simulink model "SimulModeloDinamico"  (R2015a)
settings: Solver=ode4  StartTime=0.0  StopTime=10.0  FixedStep=.001  RelTol=1e-3
libraries: dspinverses x1
settings Model: Creator=Sala6  LastModifiedBy=Sala1

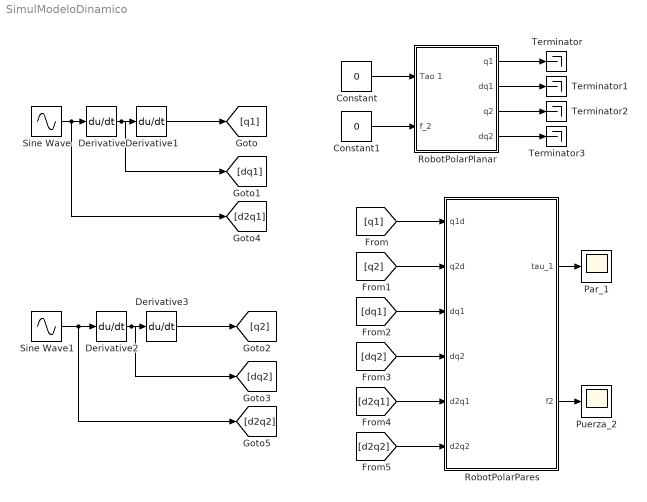
== system SimulModeloDinamico ==
  Constant : Constant  Value=0
  Constant1 : Constant  Value=0
  Derivative{,1..3} (4 alike) : Derivative
  "Par_1 " : Scope
  Puerza_2 : Scope
  RobotPolarPares : Subsystem  mask{m1=.2, m2=.1, l1=.15, lc1=.075, lc2=.05, I1z=.002, I2z=.001, g=9.81, q1_0=pi/3, dq1_0=0, q2_0=.15, dq2_0=0}
      mask prompts: m1 "Masa Eslabon1"; m2 "Masa Eslabon2"; l1 "Longitud Eslabon1"; lc1 "Longitud al Centro de Masa 1"; lc2 "Longitud al Centro de Masa 1"; I1z "Momento de Inercia Eslabon 1"; I2z "Momento de Inercia Eslabon 2"; g "Constante de Gravedad (g)"; q1_0 "Posicion inicial eslabon 1"; dq1_0 "Velocidad inicial eslabon 1"; q2_0 "Posicion inicial eslabon 2"; dq2_0 "Velocidad inicial eslabon 1"
  RobotPolarPlanar : Subsystem  mask{m1=.2, m2=.1, l1=.15, lc1=.075, lc2=.05, I1z=.002, I2z=.001, g=9.81, q1_0=pi/3, dq1_0=0, q2_0=.15, dq2_0=0}
      mask prompts: m1 "Masa Eslabon1"; m2 "Masa Eslabon2"; l1 "Longitud Eslabon1"; lc1 "Longitud al Centro de Masa 1"; lc2 "Longitud al Centro de Masa 1"; I1z "Momento de Inercia Eslabon 1"; I2z "Momento de Inercia Eslabon 2"; g "Constante de Gravedad (g)"; q1_0 "Posicion inicial eslabon 1"; dq1_0 "Velocidad inicial eslabon 1"; q2_0 "Posicion inicial eslabon 2"; dq2_0 "Velocidad inicial eslabon 1"
  Sine Wave : Sin  Amplitude=pi/2  Frequency=4*pi  SampleTime=0
  Sine Wave1 : Sin  Amplitude=.1  Frequency=2*pi  SampleTime=0
  Terminator{,1..3} (4 alike) : Terminator
  wires:
  Sine Wave/1 -> [d2q1], Derivative/1
  Derivative/1 -> [dq1], Derivative1/1
  Derivative1/1 -> [q1]
  Sine Wave1/1 -> [d2q2], Derivative2/1
  Derivative2/1 -> Derivative3/1, [dq2]
  Derivative3/1 -> [q2]
  [q1] -> RobotPolarPares/1(q1d)
  [q2] -> RobotPolarPares/2(q2d)
  [dq1] -> RobotPolarPares/3(dq1)
  [dq2] -> RobotPolarPares/4(dq2)
  [d2q1] -> RobotPolarPares/5(d2q1)
  [d2q2] -> RobotPolarPares/6(d2q2)
  RobotPolarPares/1(tau_1) -> "Par_1 "/1
  RobotPolarPares/2(f2) -> Puerza_2/1
  RobotPolarPlanar/2(dq1) -> Terminator1/1
  RobotPolarPlanar/1(q1) -> Terminator/1
  RobotPolarPlanar/3(q2) -> Terminator2/1
  RobotPolarPlanar/4(dq2) -> Terminator3/1
  Constant/1 -> RobotPolarPlanar/1("Tao 1 ")
  Constant1/1 -> RobotPolarPlanar/2("f_2 ")

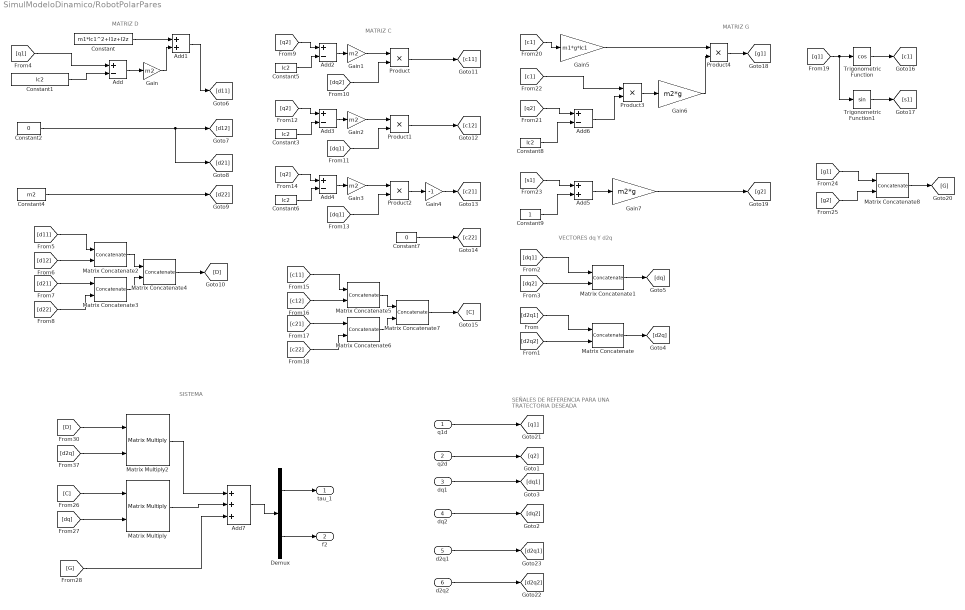
== system SimulModeloDinamico/RobotPolarPares ==
  note: SISTEMA
  note: SEÑALES DE REFERENCIA PARA UNA TRATECTORIA DESEADA
  note: MATRIZ D
  note: MATRIZ C
  note: VECTORES dq Y d2q
  note: MATRIZ G
  q1d : Inport
  q2d : Inport  Port=2
  dq1 : Inport  Port=3
  dq2 : Inport  Port=4
  d2q1 : Inport  Port=5
  d2q2 : Inport  Port=6
  Add{,2..4,6} (5 alike) : Sum  Inputs=+-
  Add1 : Sum
  Add5 : Sum
  Add7 : Sum  Inputs=+++
  Constant : Constant  Value=m1*lc1^2+I1z+I2z
  Constant{1,3,5..6,8} (5 alike) : Constant  Value=lc2
  Constant2 : Constant  Value=0
  Constant4 : Constant  Value=m2
  Constant7 : Constant  Value=0
  Constant9 : Constant
  Demux : Demux  Outputs=2
  Gain{,1..3} (4 alike) : Gain  Gain=m2
  Gain4 : Gain  Gain=-1
  Gain5 : Gain  Gain=m1*g*lc1
  Gain6 : Gain  Gain=m2*g
  Gain7 : Gain  Gain=m2*g
  Matrix Concatenate{,1,4,7..8} (5 alike) : Concatenate  Mode=Multidimensional array
  Matrix Concatenate{2..3,5..6} (4 alike) : Concatenate  Mode=Multidimensional array  ConcatenateDimension=2
  Matrix Multiply : Product  Multiplication=Matrix(*)
  Matrix Multiply2 : Product  Multiplication=Matrix(*)
  Product{,1..4} (5 alike) : Product
  Trigonometric Function : Trigonometry  Operator=cos
  Trigonometric Function1 : Trigonometry
  tau_1 : Outport
  f2 : Outport  Port=2
  wires:
  Demux/2 -> f2/1
  Demux/1 -> tau_1/1
  Add7/1 -> Demux/1
  [dq] -> Matrix Multiply/2
  [C] -> Matrix Multiply/1
  q1d/1 -> [q1]
  q2d/1 -> [q2]
  Matrix Concatenate8/1 -> [G]
  [g2] -> Matrix Concatenate8/2
  [g1] -> Matrix Concatenate8/1
  Gain7/1 -> [g2]
  Add5/1 -> Gain7/1
  Constant9/1 -> Add5/2
  [s1] -> Add5/1
  Product4/1 -> [g1]
  Gain6/1 -> Product4/2
  Gain5/1 -> Product4/1
  Product3/1 -> Gain6/1
  Add6/1 -> Product3/2
  [c1] -> Product3/1
  Constant8/1 -> Add6/2
  [q2] -> Add6/1
  [c1] -> Gain5/1
  Trigonometric Function1/1 -> [s1]
  Trigonometric Function/1 -> [c1]
  [q1] -> Trigonometric Function/1, Trigonometric Function1/1
  Matrix Concatenate6/1 -> Matrix Concatenate7/2
  Matrix Concatenate5/1 -> Matrix Concatenate7/1
  [c12] -> Matrix Concatenate5/2
  [c22] -> Matrix Concatenate6/2
  [c21] -> Matrix Concatenate6/1
  Matrix Concatenate7/1 -> [C]
  [c11] -> Matrix Concatenate5/1
  Constant7/1 -> [c22]
  Gain4/1 -> [c21]
  Product2/1 -> Gain4/1
  [dq1] -> Product2/2
  Gain3/1 -> Product2/1
  Add4/1 -> Gain3/1
  Constant6/1 -> Add4/2
  [q2] -> Add4/1
  Product1/1 -> [c12]
  [dq1] -> Product1/2
  Gain2/1 -> Product1/1
  Add3/1 -> Gain2/1
  Constant3/1 -> Add3/2
  [q2] -> Add3/1
  Product/1 -> [c11]
  [dq2] -> Product/2
  Gain1/1 -> Product/1
  Add2/1 -> Gain1/1
  Constant5/1 -> Add2/2
  [q2] -> Add2/1
  Matrix Concatenate3/1 -> Matrix Concatenate4/2
  Matrix Concatenate2/1 -> Matrix Concatenate4/1
  [d12] -> Matrix Concatenate2/2
  [d22] -> Matrix Concatenate3/2
  [d21] -> Matrix Concatenate3/1
  Matrix Concatenate4/1 -> [D]
  [d11] -> Matrix Concatenate2/1
  Constant4/1 -> [d22]
  Constant2/1 -> [d12], [d21]
  Add1/1 -> [d11]
  Gain/1 -> Add1/2
  Constant/1 -> Add1/1
  Add/1 -> Gain/1
  Constant1/1 -> Add/2
  [q1] -> Add/1
  Matrix Concatenate1/1 -> [dq]
  Matrix Concatenate/1 -> [d2q]
  [dq2] -> Matrix Concatenate1/2
  [dq1] -> Matrix Concatenate1/1
  [d2q2] -> Matrix Concatenate/2
  [d2q1] -> Matrix Concatenate/1
  [d2q] -> Matrix Multiply2/2
  [D] -> Matrix Multiply2/1
  Matrix Multiply2/1 -> Add7/1
  Matrix Multiply/1 -> Add7/2
  [G] -> Add7/3
  dq1/1 -> [dq1]
  dq2/1 -> [dq2]
  d2q1/1 -> [d2q1]
  d2q2/1 -> [d2q2]

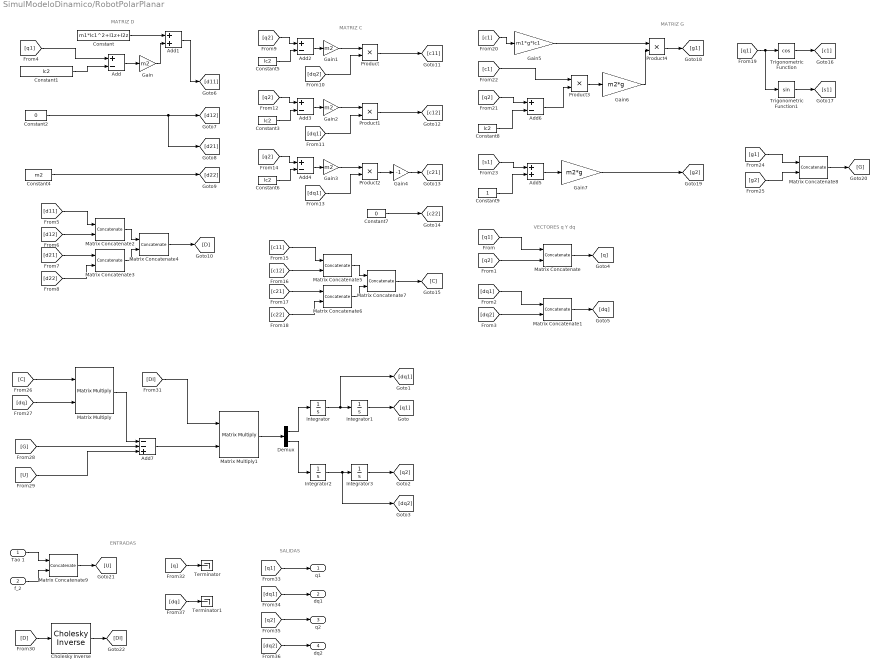
== system SimulModeloDinamico/RobotPolarPlanar ==
  note: ENTRADAS
  note: SALIDAS
  note: MATRIZ G
  note: VECTORES q Y dq
  note: MATRIZ C
  note: MATRIZ D
  "Tao 1 " : Inport
  "f_2 " : Inport  Port=2
  Add{,2..4,6} (5 alike) : Sum  Inputs=+-
  Add1 : Sum
  Add5 : Sum
  Add7 : Sum  Inputs=--+
  Cholesky Inverse : dspinverses/Cholesky Inverse  errmode=Warning
  Constant : Constant  Value=m1*lc1^2+I1z+I2z
  Constant{1,3,5..6,8} (5 alike) : Constant  Value=lc2
  Constant2 : Constant  Value=0
  Constant4 : Constant  Value=m2
  Constant7 : Constant  Value=0
  Constant9 : Constant
  Demux : Demux  Outputs=2
  Gain{,1..3} (4 alike) : Gain  Gain=m2
  Gain4 : Gain  Gain=-1
  Gain5 : Gain  Gain=m1*g*lc1
  Gain6 : Gain  Gain=m2*g
  Gain7 : Gain  Gain=m2*g
  Integrator : Integrator  InitialCondition=dq1_0
  Integrator1 : Integrator  InitialCondition=q1_0
  Integrator2 : Integrator  InitialCondition=dq2_0
  Integrator3 : Integrator  InitialCondition=q2_0
  Matrix Concatenate{,1,4,7..9} (6 alike) : Concatenate  Mode=Multidimensional array
  Matrix Concatenate{2..3,5..6} (4 alike) : Concatenate  Mode=Multidimensional array  ConcatenateDimension=2
  Matrix Multiply : Product  Multiplication=Matrix(*)
  Matrix Multiply1 : Product  Multiplication=Matrix(*)
  Product{,1..4} (5 alike) : Product
  Terminator : Terminator
  Terminator1 : Terminator
  Trigonometric Function : Trigonometry  Operator=cos
  Trigonometric Function1 : Trigonometry
  q1 : Outport
  dq1 : Outport  Port=2
  q2 : Outport  Port=3
  dq2 : Outport  Port=4
  wires:
  [q1] -> q1/1
  [dq1] -> dq1/1
  [q2] -> q2/1
  Integrator/1 -> [dq1], Integrator1/1
  Integrator2/1 -> [dq2], Integrator3/1
  Integrator1/1 -> [q1]
  Integrator3/1 -> [q2]
  [q1] -> Matrix Concatenate/1
  [q2] -> Matrix Concatenate/2
  [dq1] -> Matrix Concatenate1/1
  [dq2] -> Matrix Concatenate1/2
  Matrix Concatenate/1 -> [q]
  Matrix Concatenate1/1 -> [dq]
  [q1] -> Add/1
  Constant1/1 -> Add/2
  Add/1 -> Gain/1
  Constant/1 -> Add1/1
  Gain/1 -> Add1/2
  Add1/1 -> [d11]
  Constant2/1 -> [d21], [d12]
  Constant4/1 -> [d22]
  [d11] -> Matrix Concatenate2/1
  Matrix Concatenate4/1 -> [D]
  [d21] -> Matrix Concatenate3/1
  [d22] -> Matrix Concatenate3/2
  [d12] -> Matrix Concatenate2/2
  Matrix Concatenate2/1 -> Matrix Concatenate4/1
  Matrix Concatenate3/1 -> Matrix Concatenate4/2
  [q2] -> Add2/1
  Constant5/1 -> Add2/2
  Add2/1 -> Gain1/1
  Gain1/1 -> Product/1
  [dq2] -> Product/2
  Product/1 -> [c11]
  [q2] -> Add3/1
  Constant3/1 -> Add3/2
  Add3/1 -> Gain2/1
  Gain2/1 -> Product1/1
  [dq1] -> Product1/2
  Product1/1 -> [c12]
  [q2] -> Add4/1
  Constant6/1 -> Add4/2
  Add4/1 -> Gain3/1
  Gain3/1 -> Product2/1
  [dq1] -> Product2/2
  Product2/1 -> Gain4/1
  Gain4/1 -> [c21]
  Constant7/1 -> [c22]
  [c11] -> Matrix Concatenate5/1
  Matrix Concatenate7/1 -> [C]
  [c21] -> Matrix Concatenate6/1
  [c22] -> Matrix Concatenate6/2
  [c12] -> Matrix Concatenate5/2
  Matrix Concatenate5/1 -> Matrix Concatenate7/1
  Matrix Concatenate6/1 -> Matrix Concatenate7/2
  [q1] -> Trigonometric Function1/1, Trigonometric Function/1
  Trigonometric Function/1 -> [c1]
  Trigonometric Function1/1 -> [s1]
  [c1] -> Gain5/1
  [q2] -> Add6/1
  Constant8/1 -> Add6/2
  [c1] -> Product3/1
  Add6/1 -> Product3/2
  Product3/1 -> Gain6/1
  Gain5/1 -> Product4/1
  Gain6/1 -> Product4/2
  Product4/1 -> [g1]
  [s1] -> Add5/1
  Constant9/1 -> Add5/2
  Add5/1 -> Gain7/1
  Gain7/1 -> [g2]
  [g1] -> Matrix Concatenate8/1
  [g2] -> Matrix Concatenate8/2
  Matrix Concatenate8/1 -> [G]
  "Tao 1 "/1 -> Matrix Concatenate9/1
  "f_2 "/1 -> Matrix Concatenate9/2
  Matrix Concatenate9/1 -> [U]
  [C] -> Matrix Multiply/1
  [dq] -> Matrix Multiply/2
  Matrix Multiply/1 -> Add7/1
  [G] -> Add7/2
  [U] -> Add7/3
  [D] -> Cholesky Inverse/1
  Cholesky Inverse/1 -> [DI]
  Add7/1 -> Matrix Multiply1/2
  [DI] -> Matrix Multiply1/1
  Matrix Multiply1/1 -> Demux/1
  Demux/1 -> Integrator/1
  Demux/2 -> Integrator2/1
  [q] -> Terminator/1
  [dq2] -> dq2/1
  [dq] -> Terminator1/1
